simulink model "speed"  (R2018b)
settings: Solver=FixedStepAuto  StartTime=0.0  StopTime=inf  FixedStep=0.01  RelTol=1e-3  EnableMultiTasking=on
libraries: arduinolib x4, simulink x1
settings Model: ExtModeTrigDuration=2  Creator=Legion  LastModifiedBy=Rama2
settings DataIOCC: ReturnWorkspaceOutputs=on
settings OptimizationCC: EnhancedBackFolding=on  PassReuseOutputArgsAs=Individual arguments  ZeroExternalMemoryAtStartup=off  ZeroInternalMemoryAtStartup=off  MaxStackSize=64  OptimizeBlockOrder=speed  DifferentSizesBufferReuse=on  OptimizationCustomize=off
settings DebuggingCC: ParameterTunabilityLossMsg=error
settings HardwareCC: ProdBitPerInt=16  ProdBitPerPointer=16  ProdBitPerSizeT=16  ProdBitPerPtrDiffT=16  ProdLargestAtomicFloat=None  ProdWordSize=8  ProdHWDeviceType=Atmel->AVR
settings SFSimCC: MATLABDynamicMemAlloc=off
settings RTWCC: SystemTargetFile=ert.tlc  HardwareBoard=Arduino Uno  TemplateMakefile=ert_default_tmf  GenerateReport=on  Toolchain=Arduino AVR  BuildConfiguration=Faster Runs  IncludeHyperlinkInReport=on  LaunchReport=on  GenerateTraceInfo=on  GenerateTraceReport=on  GenerateTraceReportSl=on  GenerateTraceReportSf=on  GenerateTraceReportEml=on
settings CodeAppCC: ForceParamTrailComments=on  IgnoreCustomStorageClasses=off  OperatorAnnotations=on  SimulinkDataObjDesc=on  SFDataObjDesc=on  InsertBlockDesc=on
settings ERTTargetCC: SupportContinuousTime=on  SupportVariableSizeSignals=on  ExtModeStaticAllocSize=2048

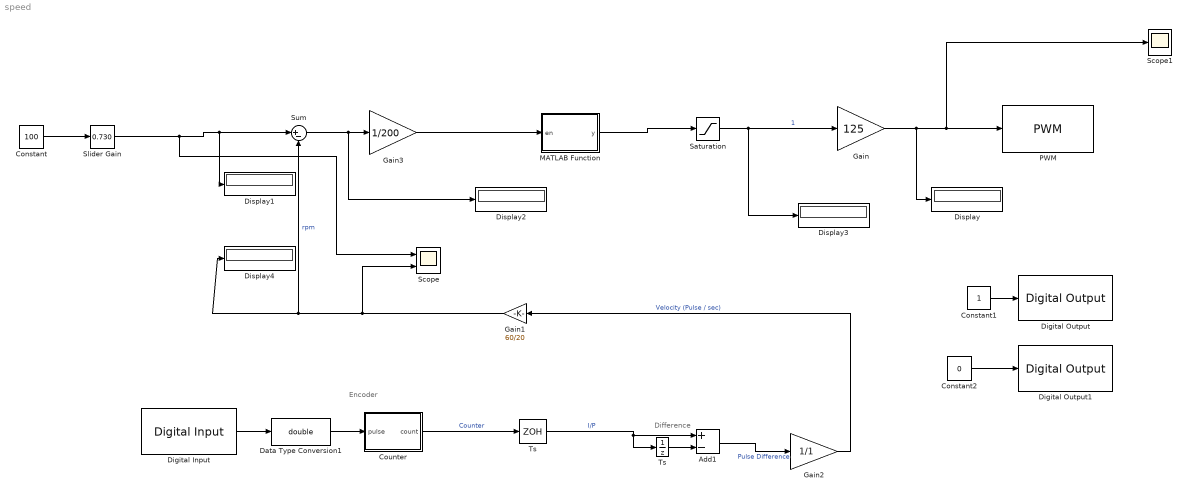
== system speed ==
  note: Encoder
  note: Difference
  Add1 : Sum  Inputs=+-
  Constant : Constant  Value=100
  Constant1 : Constant
  Constant2 : Constant  Value=0
  Counter : MATLAB Function  TreatAsAtomicUnit=on
  Data Type Conversion1 : DataTypeConversion  OutDataTypeStr=double
  Digital Input : arduinolib/Digital Input  pinNumber=7  sampleTime=0.01  blockPlatform=arduino
      settings: SourceProductName=Simulink Support Package for Arduino Hardware
  Digital Output : arduinolib/Digital Output  pinNumber=8  blockPlatform=arduino
  Digital Output1 : arduinolib/Digital Output  pinNumber=9  blockPlatform=arduino
  Display{,1..4} (5 alike) : Display
  Gain : Gain  Gain=125
  Gain1 : Gain  Gain=60/20
  Gain2 : Gain  Gain=1/1
  Gain3 : Gain  Gain=1/200
  MATLAB Function : MATLAB Function  TreatAsAtomicUnit=on
  PWM : arduinolib/PWM  pinNumber=5  EnableInputFrequency=off  InitialFrequency=2000  InitialDutyCycle=0  NotificationType=None  blockPlatform=arduino
  Saturation : Saturate  UpperLimit=1  LowerLimit=0
  Scope : Scope  NumInputPorts=2
  Scope1 : Scope
  Slider Gain : simulink/Math Operations/Slider Gain  gain=0.730  low=0  high=1
  Sum : Sum  Inputs=|+-
  "Ts " : ZeroOrderHold
  "Ts  " : UnitDelay
  wires:
  Sum/1 -> Display2/1, Gain3/1
  "Ts "/1 -> Add1/1, "Ts  "/1  "I/P"
  Digital Input/1 -> Data Type Conversion1/1
  Counter/1(count) -> "Ts "/1  "Counter"
  Data Type Conversion1/1 -> Counter/1(pulse)
  "Ts  "/1 -> Add1/2
  Add1/1 -> Gain2/1  "Pulse Difference"
  Gain2/1 -> Gain1/1  "Velocity (Pulse / sec)"
  Saturation/1 -> Display3/1, Gain/1  "1"
  Constant1/1 -> Digital Output/1
  Constant2/1 -> Digital Output1/1
  Gain/1 -> Display/1, Scope1/1, PWM/1
  Constant/1 -> Slider Gain/1
  Slider Gain/1 -> Scope/1, Display1/1, Sum/1
  Gain1/1 -> Scope/2, Display4/1, Sum/2  "rpm"
  Gain3/1 -> MATLAB Function/1(en)
  MATLAB Function/1(y) -> Saturation/1

== matlab function speed/MATLAB Function ==
  data: en input; y output
function y = fcn(en)
persistent kp ki ts eo io
if isempty(io)
    io=0;
    eo=1;
    kp=5;
    ki=0.1;
    ts=1;
end 
io=io+(ts*eo)
y=(kp*en)+(ki*io)
eo=en


end

== matlab function speed/Counter ==
  data: pulse input; count output
function count = countup(pulse)
    persistent c p
    if isempty(c)
        c = 0;
        p = 0;
    end
    if (p == 0 && pulse == 1)
       c = c+1; 
    end
    p = pulse;
    count = c ;
end
